simulink model "epex10Diagram"  (R2021a)
settings: Solver=FixedStepAuto  StartTime=0.0  StopTime=100  FixedStep=0.5  RelTol=1e-3
values from neighbouring files (symbols this model uses):
  a = [-1.6065;0.6065]    [epex10_1.m]    (also in epex4_1.m; epex5_1.m; epex6_1.m = 1; epex7_2.m)
  am = [-1.3205;0.4966]    [epex10_1.m]    (also in epex4_1.m; epex5_1.m; epex7_2.m; epex9_1.m)
  b = [0.1065;0.0902]    [epex10_1.m]    (also in epex4_1.m; epex5_1.m; epex6_1.m = 1; epex7_2.m)
  bm = beta*b    [epex10_1.m]    (also in epex4_1.m = [0.1761;0]; epex5_1.m; epex7_2.m = [0.1761;0]; epex9_1.m)
  S0 = b(2)*(a0*am(1)-a(2)-am(1)*a(1)+a(1)^2+am(2)-a(1)*a0)/(b(2)^2-a(1)*b(1)*b(2)+a(2)*b(1)^2)+      b(1)*(am(1)*a(2)-a(1)*a(2)-a0*am(2)+a0*a(2))/(b(2)^2-a(1)*b(1)*b(2)+a(2)*b(1)^2)    [epex10_1.m]    (also in epex4_1.m = (am(1)-a(1))/b(1); epex5_1.m; epex7_2.m = (am(1)-a(1))/b(1); epex9_1.m)
  S1 = b(2)*(a(1)*a(2)-am(1)*a(2)+a0*am(2)-a0*a(2))/(b(2)^2-a(1)*b(1)*b(2)+a(2)*b(1)^2)+      b(1)*(a(2)*am(2)-a(2)^2-a0*am(2)*a(1)+a0*a(2)*am(1))/(b(2)^2-a(1)*b(1)*b(2)+a(2)*b(1)^2)    [epex10_1.m]    (also in epex4_1.m = (am(2)-a(2))/b(1); epex5_1.m; epex7_2.m = (am(2)-a(2))/b(1); epex9_1.m)
  Y0 = -(1+R1)/(b(1)+b(2))    [epex10_1.m]
settings Model: Creator=dbnun  LastModifiedBy=dbnun

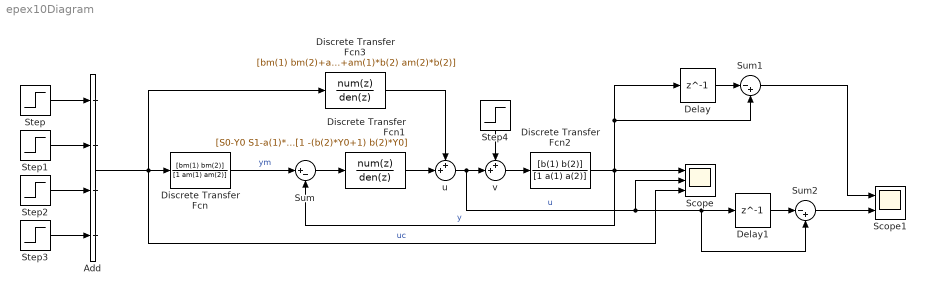
== system epex10Diagram ==
  Add : Sum  Inputs=++++
  Delay : Delay  DelayLength=1
  Delay1 : Delay  DelayLength=1
  Discrete Transfer Fcn : DiscreteTransferFcn  Numerator=[bm(1) bm(2)]  Denominator=[1 am(1) am(2)]  SampleTime=0.5
  Discrete Transfer Fcn1 : DiscreteTransferFcn  Numerator=[S0-Y0 S1-a(1)*Y0 -a(2)*Y0]  Denominator=[1 -(b(2)*Y0+1) b(2)*Y0]
  Discrete Transfer Fcn2 : DiscreteTransferFcn  Numerator=[b(1) b(2)]  Denominator=[1 a(1) a(2)]
  Discrete Transfer Fcn3 : DiscreteTransferFcn  Numerator=[bm(1) bm(2)+a(1)*bm(1) a(1)*bm(2)+a(2)*bm(1) a(2)*bm(2)]  Denominator=[b(1) b(2)+b(1)*am(1) am(2)*b(1)+am(1)*b(2) am(2)*b(2)]
  Scope : Scope  NumInputPorts=3
  Scope1 : Scope  NumInputPorts=2
  Step : Step  Time=0  SampleTime=0
  Step1 : Step  Time=25  After=-2  SampleTime=0
  Step2 : Step  Time=50  After=2  SampleTime=0
  Step3 : Step  Time=75  After=-2  SampleTime=0
  Step4 : Step  Time=40  After=0.5  SampleTime=0
  Sum : Sum  Inputs=|+-
  Sum1 : Sum  Inputs=|-+
  Sum2 : Sum  Inputs=|-+
  u : Sum  Inputs=++|
  v : Sum  Inputs=++|
  wires:
  Step2/1 -> Add/3
  Step1/1 -> Add/2
  Add/1 -> Scope/3, Discrete Transfer Fcn3/1, Discrete Transfer Fcn/1  "uc"
  Step/1 -> Add/1
  Step3/1 -> Add/4
  Discrete Transfer Fcn/1 -> Sum/1  "ym"
  Sum/1 -> Discrete Transfer Fcn1/1
  Discrete Transfer Fcn1/1 -> u/2
  u/1 -> Scope/2, Sum2/2, Delay1/1, v/2  "u"
  Discrete Transfer Fcn2/1 -> Sum1/2, Delay/1, Scope/1, Sum/2  "y"
  Discrete Transfer Fcn3/1 -> u/1
  v/1 -> Discrete Transfer Fcn2/1
  Step4/1 -> v/1
  Delay/1 -> Sum1/1
  Delay1/1 -> Sum2/1
  Sum1/1 -> Scope1/1
  Sum2/1 -> Scope1/2
